simulink model "Exercise_4_Simulink"  (R2024b)
settings: Solver=VariableStepAuto  StartTime=0.0  StopTime=10.0  RelTol=1e-3
undefined symbols (not defined in the file): k_1, k_2, k_3, q_f, T_s
libraries: robotmobilelib x1
settings Model: Creator=monet  LastModifiedBy=monet

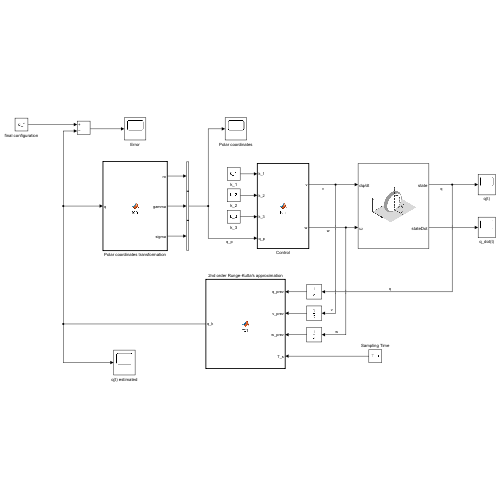
[thumbnail: Simulink's stored preview of the top-level diagram]
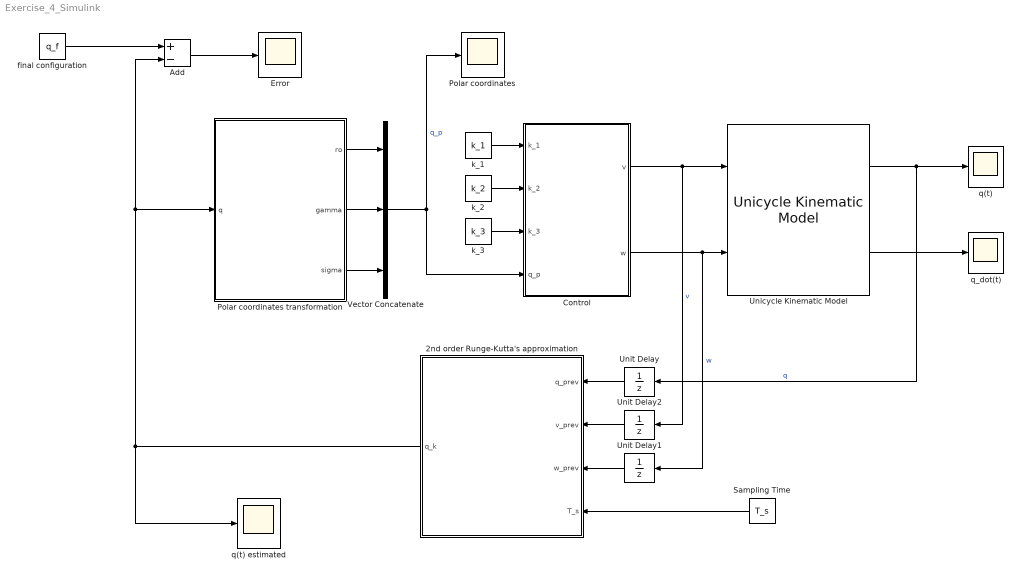
== system Exercise_4_Simulink ==
  2nd order Runge-Kutta's approximation : MATLAB Function  TreatAsAtomicUnit=on
  Add : Sum  Inputs=+-
  Control : MATLAB Function  TreatAsAtomicUnit=on
  Error : Scope
  Polar coordinates : Scope
  Polar coordinates transformation : MATLAB Function  TreatAsAtomicUnit=on
  Sampling Time : Constant  Value=T_s
  Unicycle Kinematic Model : robotmobilelib/Unicycle Kinematic Model  VehicleInputs=Wheel Speed & Heading Angular Velocity  WheelRadius=0.1  WheelSpeedRange=[-Inf Inf]  InitialState=q_i  SimulateUsing=Interpreted execution
  Unit Delay : UnitDelay  SampleTime=T_s  HasFrameUpgradeWarning=on
  Unit Delay1 : UnitDelay  SampleTime=T_s  HasFrameUpgradeWarning=on
  Unit Delay2 : UnitDelay  SampleTime=T_s  HasFrameUpgradeWarning=on
  Vector Concatenate : Concatenate  NumInputs=3
  final configuration : Constant  Value=q_f
  k_1 : Constant  Value=k_1
  k_2 : Constant  Value=k_2
  k_3 : Constant  Value=k_3
  q(t) : Scope
  q(t) estimated : Scope
  q_dot(t) : Scope
  wires:
  Unicycle Kinematic Model/1 -> Unit Delay/1, q(t)/1  "q"
  Polar coordinates transformation/1(ro) -> Vector Concatenate/1
  Polar coordinates transformation/2(gamma) -> Vector Concatenate/2
  Polar coordinates transformation/3(sigma) -> Vector Concatenate/3
  Vector Concatenate/1 -> Polar coordinates/1, Control/4(q_p)  "q_p"
  Control/1(v) -> Unit Delay2/1, Unicycle Kinematic Model/1  "v"
  Control/2(w) -> Unit Delay1/1, Unicycle Kinematic Model/2  "w"
  k_3/1 -> Control/3(k_3)
  k_2/1 -> Control/2(k_2)
  k_1/1 -> Control/1(k_1)
  Unicycle Kinematic Model/2 -> q_dot(t)/1
  Sampling Time/1 -> 2nd order Runge-Kutta's approximation/4(T_s)
  2nd order Runge-Kutta's approximation/1(q_k) -> Add/2, Polar coordinates transformation/1(q), q(t) estimated/1
  final configuration/1 -> Add/1
  Add/1 -> Error/1
  Unit Delay2/1 -> 2nd order Runge-Kutta's approximation/2(v_prev)
  Unit Delay1/1 -> 2nd order Runge-Kutta's approximation/3(w_prev)
  Unit Delay/1 -> 2nd order Runge-Kutta's approximation/1(q_prev)

== matlab function Exercise_4_Simulink/Control ==
  data: v output; w output; k_1 input; k_2 input; k_3 input; q_p input
function [v,w] = fcn(k_1,k_2,k_3,q_p)

v = k_1*q_p(1,1)*cos(q_p(2,1)); %k_1*ro*cos(gamma)
w = k_2*q_p(2,1) + k_1*sin(q_p(2,1))*cos(q_p(2,1))*(1 + k_3*q_p(3,1)/q_p(2,1));
%k_2*gamma + k_1*sin(gamma)*cos(gamma)*(1 + k_3*sigma/gamma)

end

== matlab function Exercise_4_Simulink/Polar coordinates transformation ==
  data: q input; ro output; gamma output; sigma output
function [ro,gamma,sigma] = fcn(q)

ro = sqrt(q(1,1)^2 + q(2,1)^2); % sqrt(x^2+y^2)
gamma = atan2(q(2,1),q(1,1)) - q(3,1) + pi; % atan2(y,x)-theta-pi
sigma = gamma + q(3,1); % gamma + theta

end

== matlab function Exercise_4_Simulink/2nd order Runge-Kutta's approximation ==
  data: q_prev input; v_prev input; w_prev input; q_k output; T_s input
function q_k   = fcn(q_prev,v_prev,w_prev,T_s)

x_k = q_prev(1,1) + v_prev*T_s*cos(q_prev(3,1) + 1/2*w_prev*T_s);
%x_prev + v_prev*T_s*cos(theta_prev + 1/2*w_prev*T_s)
y_k = q_prev(2,1) + v_prev*T_s*sin(q_prev(3,1) + 1/2*w_prev*T_s);
%y_prev + v_prev*T_s*sin(theta_prev + 1/2*w_prev*T_s)
theta_k = q_prev(3,1) + w_prev*T_s; %theta_k = theta_prev + w_prev*T_s;

q_k = [x_k,y_k,theta_k]';

end
